simulink model "usrp_QPSK_coarse_synch"  (R2017a)
settings: Solver=FixedStepDiscrete  StartTime=0.0  StopTime=inf  RelTol=1e-3  EnableMultiTasking=on
PreLoadFcn:
  | %%%%%%%%%%%%%%%%%%%%%%%%%%%%%%%%%%%%%%%%%%%%%%%%%%%%%%%%%%%%%%%%%%%%%%%%%%%
  | % check to see if Simulink library folder is missing from the MATLAB path %
  | %%%%%%%%%%%%%%%%%%%%%%%%%%%%%%%%%%%%%%%%%%%%%%%%%%%%%%%%%%%%%%%%%%%%%%%%%%%
  | if isempty(strfind(path, 'rtlsdr_book_library'))
  | 
  |     % create error window
  |     fig_error = figure(...
  |         'Name', 'Error: RTL-SDR Book Library',...
  |         'Toolbar','none',...
  |         'MenuBar','none',...
  |         'NumberTitle','off',...
  |         'Resize','off',...
  |         'WindowStyle','modal');
  |     fig_error.Position(3) = 600;
  |     fig_error.Position(4) = 150;
  |     fig_axes = axes(...
  |         'Parent',fig_error,...
  |         'Position',[0,0,1,1],...
  |         'visible','off');
  |     % error message
  |     t_title = text(.05,.8,...
  |         'MISSING DIRECTORIES',...
  |         'FontSize',11.5);
  |     t_body = text(.075,.6,...
  |         [{'Simulink cannot find the  \it{<root>}\rm / \it{rtlsdr\_book\_library}\rm  folder in the \it{MATLAB Path}\rm.'},...
  |         {'Please set the MATLAB path following the instructions given in Exercise 2.4.'}],...
  |         'FontSize',10.5);
  |     % buttons
  |     btn_path = uicontrol(...
  |         'Parent',fig_error,...
  |         'String','Set Path Now',...
  |         'FontSize',10,...
  |         'Callback', 'pathtool; close(fig_error);',...
  |         'Position', [fig_error.Position(3)/2-210, 30, 200, 30]);
  |     btn_abort = uicontrol(...
  |         'Parent',fig_error,...
  |         'String','No thanks',...
  |         'FontSize',10,...
  |         'Callback', 'close(fig_error); abort=1;',...
  |         'Position', [fig_error.Position(3)/2+10, 30, 200, 30]);
  | 
  |     % pause to allow user to interact with error box
  |     uiwait(fig_error);
  | 
  |     % abort simulation
  |     try
  |         if abort==1
  |             set_param(gcs, 'SimulationCommand', 'stop');
  |         end
  |     end
  | 
  |     % if user has set path, allow diagram to be updated
  |     if ~exist('abort','var')
  |         % create error window
  |         fig_update = figure(...
  |             'Name', 'Update Diagram',...
  |             'Toolbar','none',...
  |             'MenuBar','none',...
  |             'NumberTitle','off',...
  |             'Resize','off');
  |         fig_update.Position(3) = 400;
  |         fig_update.Position(4) = 120;
  |         fig_axes = axes(...
  |             'Parent',fig_update,...
  |             'Position',[0,0,1,1],...
  |             'visible','off');
  |         % instruction message
  |         t_body = text(.075,.7,...
  |             'Once you have set the path, update the block diagram',...
  |             'FontSize',10.5);
  |         % button
  |         btn_update = uicontrol(...
  |             'Parent',fig_update,...
  |             'String','Update Block Diagram',...
  |             'FontSize',10,...
  |             'Callback', 'set_param(gcs,''SimulationCommand'',''update''); close(gcf)',...
  |             'Position', [fig_update.Position(3)/2-100, 30, 200, 30]);
  |     end
  | 
  |     % clear error components
  |     clear('fig_error','fig_update','fig_axes','t_title','t_body','btn_path','btn_abort','btn_update','abort');
  | 
  | end
  | %%%%%%%%%%%%%%%%%%%%%%%%%%%%%%%%%%%%%%%%%%%%%%%%%%%%%%%%%%%%%%%%%%%%%%%%%%%
undefined symbols (not defined in the file): fdesignblkfcn, gcbh, startfcn_spectrum_analyzer
libraries: dspmlti4 x3, commrandsrc2 x1, rtlsdr_book_library x1, commdigbbndpm3 x1, commfilt2 x1, commsdrhw_v2 x1
CloseFcn:
  | closefcn_model;
Description:
  | Software, Simulation Examples and Design Exercises Licence Agreement
  | 
  | This license agreement refers to the simulation examples, design exercises and files,
  | and associated software MATLAB and Simulink resources that accompany the book:
  | 
  |      Title: Software Defined Radio using MATLAB & Simulink and the RTL-SDR
  |      Published by Strathclyde Academic Media, 2015
  |      Authored by Robert W. Stewart, Kenneth W. Barlee, Dale S.W. Atkinson,
  |      and Louise H. Crockett
  | 
  | and made available as a download from, www.desktopSDR.com or variously acquired
  | by other means such as via USB storage, cloud storage, disk or any other electronic
  | or optical or magnetic storage mechanism. These files and associated software may
  | be used subject to the terms of agreement of the conditions below:
  | 
  |     Copyright © 2015 Robert W. Stewart, Kenneth W. Barlee, Dale S.W. Atkinson,
  |     and Louise H. Crockett
  |     All rights reserved.
  | 
  | Redistribution and use in source and binary forms, with or without modification, are
  | permitted provided that the following conditions are met:
  | 
  |    1.  Redistributions of source code must retain the above copyright notice, this list of
  |         conditions and the following disclaimer.
  | 
  |    2.  Redistributions in binary form must reproduce the above copyright notice, this
  |         list of conditions and the following disclaimer in the documentation and/or other
  |         materials provided with the distribution.
  | 
  |    3.  Neither the name of the copyright holder nor the names of its contributors may
  |         be used to endorse or promote products derived from this software without
  |         specific prior written permission.
  | 
  |    4.  In all cases, the software is, and all modifications and derivatives of the
  |         software shall be, licensed to you solely for use in conjunction with The
  |         MathWorks, Inc. products and service offerings.
  | 
  | THIS SOFTWARE IS PROVIDED BY THE COPYRIGHT HOLDERS AND CONTRIBUTORS
  | "AS IS" AND ANY EXPRESS OR IMPLIED WARRANTIES, INCLUDING, BUT NOT LIMITED
  | TO, THE IMPLIED WARRANTIES OF MERCHANTABILITY AND FITNESS FOR A
  | PARTICULAR PURPOSE ARE DISCLAIMED. IN NO EVENT SHALL THE COPYRIGHT
  | HOLDER OR CONTRIBUTORS BE LIABLE FOR ANY DIRECT, INDIRECT, INCIDENTAL,
  | SPECIAL, EXEMPLARY, OR CONSEQUENTIAL DAMAGES (INCLUDING, BUT NOT
  | LIMITED TO, PROCUREMENT OF SUBSTITUTE GOODS OR SERVICES; LOSS OF USE,
  | DATA, OR PROFITS; OR BUSINESS INTERRUPTION) HOWEVER CAUSED AND ON ANY
  | THEORY OF LIABILITY, WHETHER IN CONTRACT, STRICT LIABILITY, OR TORT
  | (INCLUDING NEGLIGENCE OR OTHERWISE) ARISING IN ANY WAY OUT OF THE USE
  | OF THIS SOFTWARE, EVEN IF ADVISED OF THE POSSIBILITY OF SUCH DAMAGE.
  | 
  | 
  | Audio Tracks used in Simulations Examples and Design Exercises
  | 
  | The music and vocal files used within the Examples files and software within the book
  | were variously written, arranged, performed, recorded and produced by Garrey Rice,
  | Adam Struth, Jamie Struth, Iain Thistlethwaite and also Marshall Craigmyle who
  | collectively, and individually where appropriate, assert and retain all of their copyright,
  | performance and artistic rights. Permission to use and reproduce this music is
  | granted for all purposes associated with MATLAB and Simulink software and the
  | simulation examples and design exercises files that accompany this book. Requests to
  | use the music for any other purpose should be directed to: info@desktopSDR.com.
  | For information on music track names, full credits, and links to the musicians please
  | refer to www.desktopSDR.com/more/audio.
settings Model: SimulationMode=accelerator  Creator=desktopSDR Team  LastModifiedBy=vladi
settings DataIOCC: SaveFormat=Array  SaveOutput=off  SignalLogging=off  SaveTime=off
settings OptimizationCC: LifeSpan=inf  SimCompilerOptimization=on
settings DebuggingCC: SolverPrmCheckMsg=warning  SFUnexpectedBacktrackingDiag=warning  SFNoUnconditionalDefaultTransitionDiag=warning  SFExecutionAtInitializationDiag=none
settings HardwareCC: ProdBitPerPointer=32  ProdBitPerSizeT=32  ProdBitPerPtrDiffT=32  ProdLargestAtomicFloat=None  ProdIntDivRoundTo=Undefined  ProdEndianess=Unspecified  ProdWordSize=32  ProdHWDeviceType=32-bit Generic
settings ModelReferenceCC: PropagateSignalLabelsOutOfModel=off
settings GRTTargetCC: TargetLangStandard=C89/C90 (ANSI)  GeneratePreprocessorConditionals=Disable all
settings ConfigComp: CovMetricSettings=dw  CovHtmlReporting=on  CovSaveCumulativeToWorkspaceVar=on  CovSaveSingleToWorkspaceVar=on  CovExternalEMLEnable=off  CovSFcnEnable=off

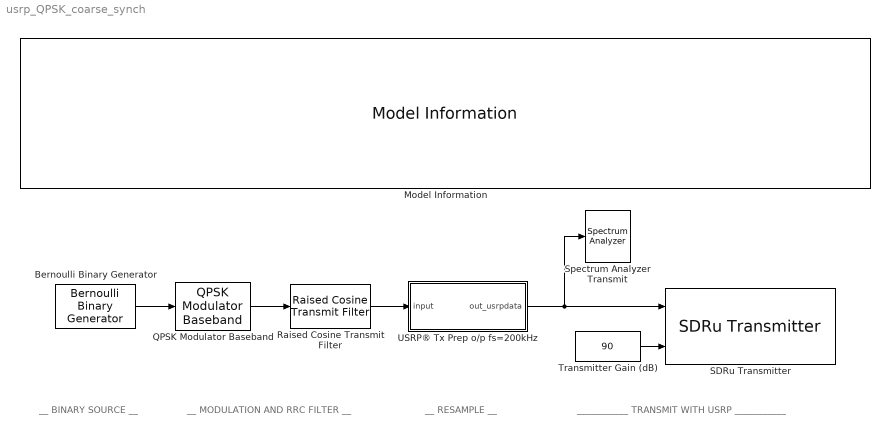
== system usrp_QPSK_coarse_synch ==
  note: __ BINARY SOURCE __
  note: __ MODULATION AND RRC FILTER __
  note: ___________ TRANSMIT WITH USRP ___________
  note: __ RESAMPLE __
  Bernoulli Binary Generator : commrandsrc2/Bernoulli Binary Generator  P=0.5  seed=61  Ts=1/2e3  frameBased=on  sampPerFrame=2  orient=off  outDataType=boolean
  Model Information : rtlsdr_book_library/Additional Tools/Model Information/Model Information
      settings: SourceProductName=RTL-SDR Book Library
  QPSK Modulator Baseband : commdigbbndpm3/QPSK Modulator Baseband  InType=Bit  Enc=Gray  Ph=pi/4  outDtype=double  outWordLen=16  outUDDataType=sfix(16)  outFracLenMode=Best precision  outFracLen=15  outDataTypeStr=double  outLastDataTypeStr=double
  Raised Cosine Transmit Filter : commfilt2/Raised Cosine Transmit Filter  filtType=Square root  R=0.5  filtSpan=12  N=4  filterGain=1  InputProcessing=Columns as channels (frame based)  RateOptions=Allow multirate processing  framing=Mute  checkCoeff=off  variableName=rcTxFilt  checkGain=Normalized  sampMode=Mute  saveAsFlag=0  currentFiltSpan=12  D=(12)/2  launchFVT=on  roundingMode=Floor  overflowMode=off  coeffDataTypeStr=Inherit: Same word length as input  coeffMin=[]  coeffMax=[]  coeffLastDataTypeStr=Inherit: Same word length as input  outputDataTypeStr=Inherit: Same as accumulator  outputMin=[]  outputMax=[]  outputLastDataTypeStr=Inherit: Same as accumulator
  SDRu Transmitter : commsdrhw_v2/SDRu Transmitter  SourceLibraryInfo="This block requires <a href=\"http://www.mathworks.com/hardware-support/usrp.html\">Communications System Toolbox Support Package for USRP Radio</a>"  rxtx=tx  platform=B210  USRP2_IP='169.254.10.2'  USRP_IP_X300='192.168.10.2'  USRP_IP_X310='192.168.10.2'  USRP_serialNumB200=''  USRP_serialNumB210='30D0D1F'  ChannelMapping=1  centerFrequency=2.484e9  centerFrequencySrc=Dialog  loOffset=0  loOffsetSrc=Dialog  PPSSource=Internal  clockSource=Internal  masterClkRateB200=32e6  masterClkRateB210=32e6  masterClkRateX300=200e6  masterClkRateX310=200e6  masterClkRateParam=32000000  gain=10  gainSrc=Input port  decimInterp=160  decimInterpSrc=Dialog  TransportDataType=int16  USRP2_IP_NUM=[51 48 68 48 68 49 70]  frameLength=362  outputDatatype=Same as transport data type  overrunUnderrunPort=off  sampleTime=1  dboardInfo=|  HOST_DATA_PORT=30000  HOST_CONTROL_PORT=30001  USRP2_DATA_PORT=32769  USRP2_CONTROL_PORT=32768  bufferMode=Continuous streaming  EnableBurstMode=off  NumFramesInBurst=100  USRP_ID='30D0D1F'
      | dbid: 0
      |           dbName: 'no db found'
      |          freqMin: 0
      |          freqMax: 0
      |          gainMin: 0
      |          gainMax: 0
      |     gainStepSize: 0
      settings: SourceProductName=Communications System Toolbox Support Package for USRP(R) Radio  SourceProductBaseCode=USRP
  Spectrum Analyzer Transmit : SpectrumAnalyzer  StartFcn=startfcn_spectrum_analyzer;
  Transmitter Gain (dB) : Constant  Value=90
  USRP® Tx Prep o/p fs=200kHz : Subsystem
  wires:
  Raised Cosine Transmit Filter/1 -> USRP® Tx Prep o/p fs=200kHz/1(input)
  Bernoulli Binary Generator/1 -> QPSK Modulator Baseband/1
  QPSK Modulator Baseband/1 -> Raised Cosine Transmit Filter/1
  USRP® Tx Prep o/p fs=200kHz/1(out_usrpdata) -> Spectrum Analyzer Transmit/1, SDRu Transmitter/1
  Transmitter Gain (dB)/1 -> SDRu Transmitter/2

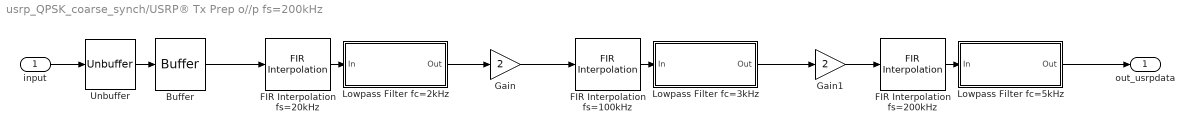
== system usrp_QPSK_coarse_synch/USRP® Tx Prep o//p fs=200kHz ==
  input : Inport
  Buffer : Buffer  N=1000
  FIR Interpolation fs=100kHz : dspmlti4/FIR Interpolation  FilterSource=Dialog parameters  h=firpm(75,[0 5e3 10e3 100e3/2]/(100e3/2), [1 1 0 0], [1 1], 20)  L=5  FilterObject=Hm_firinterp  InputProcessing=Columns as channels (frame based)  framing=Allow multirate processing  outputBufInitCond=0  roundingMode=Floor  overflowMode=off  firstCoeffDataTypeStr=Inherit: Same word length as input  firstCoeffMin=[]  firstCoeffMax=[]  firstCoeffLastDataTypeStr=Inherit: Same word length as input  outputDataTypeStr=Inherit: Same as accumulator  outputMin=[]  outputMax=[]  outputLastDataTypeStr=Inherit: Same as accumulator
      settings: SourceProductName=DSP System Toolbox
  FIR Interpolation fs=200kHz : dspmlti4/FIR Interpolation  FilterSource=Dialog parameters  h=firpm(75,[0 5e3 15e3 200e3/2]/(200e3/2), [1 1 0 0], [1 1], 20)  L=2  FilterObject=Hm_firinterp  InputProcessing=Columns as channels (frame based)  framing=Allow multirate processing  outputBufInitCond=0  roundingMode=Floor  overflowMode=off  firstCoeffDataTypeStr=Inherit: Same word length as input  firstCoeffMin=[]  firstCoeffMax=[]  firstCoeffLastDataTypeStr=Inherit: Same word length as input  outputDataTypeStr=Inherit: Same as accumulator  outputMin=[]  outputMax=[]  outputLastDataTypeStr=Inherit: Same as accumulator
      settings: SourceProductName=DSP System Toolbox
  FIR Interpolation fs=20kHz : dspmlti4/FIR Interpolation  FilterSource=Dialog parameters  h=firpm(75,[0 1.5e3 2e3 20e3/2]/(20e3/2), [1 1 0 0], [1 1], 20)  L=5  FilterObject=Hm_firinterp  InputProcessing=Columns as channels (frame based)  framing=Allow multirate processing  outputBufInitCond=0  roundingMode=Floor  overflowMode=off  firstCoeffDataTypeStr=Inherit: Same word length as input  firstCoeffMin=[]  firstCoeffMax=[]  firstCoeffLastDataTypeStr=Inherit: Same word length as input  outputDataTypeStr=Inherit: Same as accumulator  outputMin=[]  outputMax=[]  outputLastDataTypeStr=Inherit: Same as accumulator
      settings: SourceProductName=DSP System Toolbox
  Gain : Gain  Gain=2
  Gain1 : Gain  Gain=2
  Lowpass Filter fc=2kHz : Subsystem  DialogController=fdesignblkfcn  InitFcn=fdesignblkfcn(gcbh, {'InitFcn'});  mask(Lowpass Filter){}
      mask help: Design a lowpass filter
      settings: CopyFcn=fdesignblkfcn(gcbh, {'CopyFcn'});
      mask Help: helpview(mapfilelocation('dsp'), 'dsplowpassfilter');
      mask Display: disp('Lowpass')
  Lowpass Filter fc=3kHz : Subsystem  DialogController=fdesignblkfcn  InitFcn=fdesignblkfcn(gcbh, {'InitFcn'});  mask(Lowpass Filter){}
      mask help: Design a lowpass filter
      settings: CopyFcn=fdesignblkfcn(gcbh, {'CopyFcn'});
      mask Help: helpview(mapfilelocation('dsp'), 'dsplowpassfilter');
      mask Display: disp('Lowpass')
  Lowpass Filter fc=5kHz : Subsystem  DialogController=fdesignblkfcn  InitFcn=fdesignblkfcn(gcbh, {'InitFcn'});  mask(Lowpass Filter){}
      mask help: Design a lowpass filter
      settings: CopyFcn=fdesignblkfcn(gcbh, {'CopyFcn'});
      mask Help: helpview(mapfilelocation('dsp'), 'dsplowpassfilter');
      mask Display: disp('Lowpass')
  Unbuffer : Unbuffer
  out_usrpdata : Outport
  wires:
  Lowpass Filter fc=2kHz/1(Out) -> Gain/1
  Gain1/1 -> FIR Interpolation fs=200kHz/1
  Lowpass Filter fc=5kHz/1(Out) -> out_usrpdata/1
  FIR Interpolation fs=200kHz/1 -> Lowpass Filter fc=5kHz/1(In)
  Lowpass Filter fc=3kHz/1(Out) -> Gain1/1
  Gain/1 -> FIR Interpolation fs=100kHz/1
  FIR Interpolation fs=20kHz/1 -> Lowpass Filter fc=2kHz/1(In)
  FIR Interpolation fs=100kHz/1 -> Lowpass Filter fc=3kHz/1(In)
  Buffer/1 -> FIR Interpolation fs=20kHz/1
  input/1 -> Unbuffer/1
  Unbuffer/1 -> Buffer/1

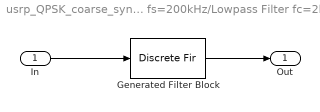
== system usrp_QPSK_coarse_synch/USRP® Tx Prep o//p fs=200kHz/Lowpass Filter fc=2kHz ==
  In : Inport
  Generated Filter Block : DiscreteFir  Tag=BlockMethodSubSystem  Coefficients=[0.0021847519133281115 -0.00063638716804181655 -0.0023212660103241909 -0.003684703237659198 -0.0032014602773711327 -0.00022955581090621909 0.0041142953344396891 0.0071385325992800097 0.0060707131982534242 0.0001440414766327583 -0.0080999805930590443 -0.013521817362168122 -0.011237343036911934 -0.00019727061121426758 0.014813892101174453 0.024611303196966375 0.020483272658574102 0.00022234086757833875 -0.028240467793545197 -0.048446158085878523 -0.042440020759801932 -0.00024042384287604289 0.07317974748482596 0.15757355588781313 0.22469386578041783 0.25024867725231437 0.22469386578041783 0.15757355588781313 0.07317974748482596 -0.00024042384287604289 -0.042440020759801932 -0.048446158085878523 -0.028240467793545197 0.00022234086757833875 0.020483272658574102 0.024611303196966375 0.014813892101174453 -0.00019727061121426758 -0.011237343036911934 -0.013521817362168122 -0.0080999805930590443 0.0001440414766327583 0.0060707131982534242 0.0071385325992800097 0.0041142953344396891 -0.00022955581090621909 -0.0032014602773711327 -0.003684703237659198 -0.0023212660103241909 -0.00063638716804181655 0.0021847519133281115]  InputProcessing=Columns as channels (frame based)
  Out : Outport
  wires:
  In/1 -> Generated Filter Block/1
  Generated Filter Block/1 -> Out/1

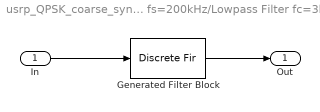
== system usrp_QPSK_coarse_synch/USRP® Tx Prep o//p fs=200kHz/Lowpass Filter fc=3kHz ==
  In : Inport
  Generated Filter Block : DiscreteFir  Tag=BlockMethodSubSystem  Coefficients=[-0.00057515568507520722 -0.00026593192242688678 -9.4236020237540661e-06 0.00055892189900990448 0.0014255273800854789 0.0024583717859701293 0.0033936724710209826 0.003860755054792385 0.0034511891942068953 0.0018255550166671136 -0.0011586820489855436 -0.0053300501670516288 -0.010129080805802448 -0.0146079399898196 -0.017519741488494139 -0.017499414997537186 -0.013311454016181199 -0.0041217984057762697 0.010264080253503808 0.029249165061641925 0.051423772534618918 0.074694530637538711 0.096555640146205129 0.11445396342826282 0.12618965566692111 0.13027622076528664 0.12618965566692111 0.11445396342826282 0.096555640146205129 0.074694530637538711 0.051423772534618918 0.029249165061641925 0.010264080253503808 -0.0041217984057762697 -0.013311454016181199 -0.017499414997537186 -0.017519741488494139 -0.0146079399898196 -0.010129080805802448 -0.0053300501670516288 -0.0011586820489855436 0.0018255550166671136 0.0034511891942068953 0.003860755054792385 0.0033936724710209826 0.0024583717859701293 0.0014255273800854789 0.00055892189900990448 -9.4236020237540661e-06 -0.00026593192242688678 -0.00057515568507520722]  InputProcessing=Columns as channels (frame based)
  Out : Outport
  wires:
  In/1 -> Generated Filter Block/1
  Generated Filter Block/1 -> Out/1

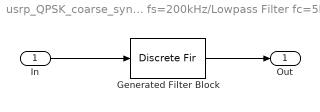
== system usrp_QPSK_coarse_synch/USRP® Tx Prep o//p fs=200kHz/Lowpass Filter fc=5kHz ==
  In : Inport
  Generated Filter Block : DiscreteFir  Tag=BlockMethodSubSystem  Coefficients=[0.0030859939042232826 0.0021255229451968799 0.0024065332531031619 0.0023002153988581349 0.0016663671617756341 0.0004165666862569549 -0.001465185986943915 -0.0038864134225252743 -0.0066439540551720367 -0.0094145602906065828 -0.011777325079299739 -0.01323929632407019 -0.013294693176780843 -0.011475658620718943 -0.0074207886249491239 -0.00092477027327775513 0.008004491255857657 0.019125597998939668 0.031955042981664794 0.045803346095610625 0.05981558768355448 0.07304915324903187 0.084551052336133248 0.093468017669346495 0.099116878346833415 0.10104623748124383 0.099116878346833415 0.093468017669346495 0.084551052336133248 0.07304915324903187 0.05981558768355448 0.045803346095610625 0.031955042981664794 0.019125597998939668 0.008004491255857657 -0.00092477027327775513 -0.0074207886249491239 -0.011475658620718943 -0.013294693176780843 -0.01323929632407019 -0.011777325079299739 -0.0094145602906065828 -0.0066439540551720367 -0.0038864134225252743 -0.001465185986943915 0.0004165666862569549 0.0016663671617756341 0.0023002153988581349 0.0024065332531031619 0.0021255229451968799 0.0030859939042232826]  InputProcessing=Columns as channels (frame based)
  Out : Outport
  wires:
  Generated Filter Block/1 -> Out/1
  In/1 -> Generated Filter Block/1
